simulink model "CLLLC_Plant_vLoad_V2"  (R2022a)
settings: Solver=FixedStepDiscrete  StartTime=0.0  StopTime=0.5  FixedStep=Step_Rate  RelTol=1e-3
model workspace (MAT data in the model file):
  CVI_INit = 0
  Fsw = Simulink.Signal
  Fsw.DataType = 'double'
  Fsw.Dimensions = -1
  Fsw.DimensionsMode = 'auto'
  Fsw.Complexity = 'auto'
  Fsw.SampleTime = -1
  Fsw.SamplingMode = 'auto'
  Fsw.InitialValue = 'fsw'
  L_Lim = 0.6
  fnerr = Simulink.Signal
  fnerr.DataType = 'double'
  fnerr.Dimensions = 1
  fnerr.DimensionsMode = 'Variable'
  fnerr.Complexity = 'auto'
  fnerr.SampleTime = -1
  fnerr.SamplingMode = 'auto'
  fsw = Simulink.Signal
  fsw.DataType = 'double'
  fsw.Dimensions = 1
  fsw.DimensionsMode = 'Variable'
  fsw.Complexity = 'auto'
  fsw.SampleTime = -1
  fsw.SamplingMode = 'auto'
  swit = Simulink.Signal
  swit.DataType = 'double'
  swit.Min = 0
  swit.Max = 1
  swit.Dimensions = -1
  swit.DimensionsMode = 'auto'
  swit.Complexity = 'auto'
  swit.SampleTime = -1
  swit.SamplingMode = 'auto'
  tsw = Simulink.Signal
  tsw.DataType = 'double'
  tsw.Dimensions = 1
  tsw.DimensionsMode = 'Variable'
  tsw.Complexity = 'auto'
  tsw.SampleTime = -1
  tsw.SamplingMode = 'auto'
values from neighbouring files (symbols this model uses):
  a0_cv_F = 0.01392699    [CLLLC_Plant_Parameters_vLoad_V2.m]
  a1_cv_F = -0.0060730    (= -0.006073)    [CLLLC_Plant_Parameters_vLoad_V2.m]
  a2_cv_F = 0.0    (= 0)    [CLLLC_Plant_Parameters_vLoad_V2.m]
  b1_cv_F = -1    [CLLLC_Plant_Parameters_vLoad_V2.m]
  b2_cv_F = 0.0    (= 0)    [CLLLC_Plant_Parameters_vLoad_V2.m]
  Cmd_Ref_Ctrl = round(Cmd_Ref * KVpri / VADC * ADCFS)    [CLLLC_Plant_Parameters_vLoad_V2.m]
  Control_Step_Rate = 50e-6    (= 5e-05)    [CLLLC_Plant_Parameters_vLoad_V2.m]
  Freq_Sw = 55.1e3    (= 55100)    [CLLLC_Plant_Parameters_vLoad_V2.m]
  KIout = 20e-3    (= 0.02)    [CLLLC_Plant_Parameters_vLoad_V2.m]
  KVpri = 0.0036102    [CLLLC_Plant_Parameters_vLoad_V2.m]
  KVsec = 0.00569815    [CLLLC_Plant_Parameters_vLoad_V2.m]
  Lm1 = Ln*LrP1    (= 8e-05)    [CLLLC_Plant_Parameters_vLoad_V2.m]
  n = 20.0/9.0    (= 2.22222222222)    [CLLLC_Plant_Parameters_vLoad_V2.m]
  R_series = 3    [CLLLC_Plant_Parameters_vLoad_V2.m]
  Reverse = 1    [CLLLC_Plant_Parameters_vLoad_V2.m]
  Step_Rate = 1e-7    (= 1e-07)    [CLLLC_Plant_Parameters_vLoad_V2.m]
  transformerCoupling = 0.999    [CLLLC_Plant_Parameters_vLoad_V2.m]
  Ts_Sw = floor(Fclk/Freq_Sw)    [CLLLC_Plant_Parameters_vLoad_V2.m]
libraries: fl_lib x36, nesl_utility x25, ee_lib x15, simulink x7, spsFirstOrderFilterLib x5, slpidlib x3, simulink_extras x3, eeGeneralControl x1
(part 1 of 3)
settings Model: Creator=siddharthaisukappal  LastModifiedBy=sgcesuser3
settings SolverCC: AlgebraicLoopSolver=TrustRegion
settings DataIOCC: ReturnWorkspaceOutputs=off
settings OptimizationCC: DefaultParameterBehavior=Inlined  UseDivisionForNetSlopeComputation=on  GainParamInheritBuiltInType=on  UseFloatMulNetSlope=on  InlineInvariantSignals=on  PassReuseOutputArgsAs=Individual arguments  ZeroExternalMemoryAtStartup=off  ZeroInternalMemoryAtStartup=off  NoFixptDivByZeroProtection=on  EfficientFloat2IntCast=on  LifeSpan=1  OptimizeBlockOrder=speed  DifferentSizesBufferReuse=on  EfficientTunableParamExpr=on
settings DebuggingCC: ParameterTunabilityLossMsg=error  UnconnectedInputMsg=warning  UnconnectedOutputMsg=warning  UnconnectedLineMsg=warning  SFMachineParentedDataDiag=warning
settings HardwareCC: ProdLongLongMode=on
settings SFSimCC: MATLABDynamicMemAlloc=off  CustomCodeUndefinedFunction=UseInterfaceOnly
settings RTWCC: SystemTargetFile=ert.tlc  TemplateMakefile=ert_default_tmf  GenerateReport=on  IncludeHyperlinkInReport=on  LaunchReport=on  GenerateTraceInfo=on  GenerateTraceReport=on  GenerateTraceReportSl=on  GenerateTraceReportSf=on  GenerateTraceReportEml=on  GenerateCodeMetricsReport=on  DLArmComputeVersion=19.05
settings CodeAppCC: ForceParamTrailComments=on  IgnoreCustomStorageClasses=off  OperatorAnnotations=on  SimulinkDataObjDesc=on  SFDataObjDesc=on  CustomSymbolStrGlobalVar=rt$N$M  CustomSymbolStrType=$N$M  CustomSymbolStrFcn=$N$M$F  CustomSymbolStrMacro=$N$M  InsertBlockDesc=on
settings ERTTargetCC: TargetLangStandard=C99 (ISO)  GenerateSampleERTMain=on  IncludeMdlTerminateFcn=off  CombineSignalStateStructs=on  SupportAbsoluteTime=off  SupportComplex=off  SupportContinuousTime=on  SupportNonInlinedSFcns=on  InlinedParameterPlacement=NonHierarchical  ERTCustomFileTemplate=example_file_process.tlc  ERTFilePackagingFormat=CompactWithDataFile
settings SimscapeCC: SimscapeLogDataHistory=20000

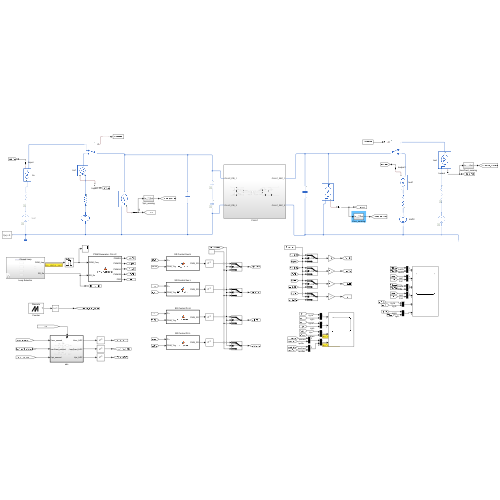
[thumbnail: Simulink's stored preview of the top-level diagram]
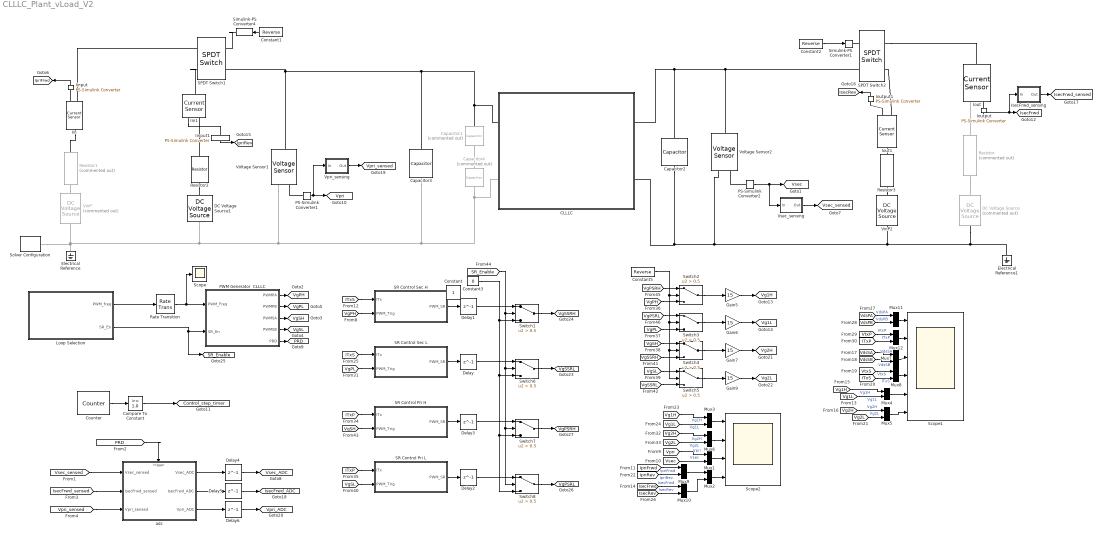
== system CLLLC_Plant_vLoad_V2 ==
  CLLLC : Subsystem
  Capacitor1 : fl_lib/Electrical/Electrical Elements/Capacitor  Commented=on  c=2800e-6 F  r=0.0496 Ohm  g=0 1/Ohm  i_specify=off  i_priority=None  i=0 A  i_nominal_specify=off  i_nominal_unit=A  i_nominal_value=1  v_specify=off  v_priority=None  v=390 V  v_nominal_specify=off  v_nominal_unit=V  v_nominal_value=1  vc_specify=on  vc_priority=High  vc=403 V  vc_nominal_specify=off  vc_nominal_unit=V  vc_nominal_value=1
      settings: SourceProductBaseCode=PW,SS,VE
  Capacitor2 : fl_lib/Electrical/Electrical Elements/Capacitor  c=50e-6 F  r=9.5e-3 Ohm  g=0 1/Ohm  i_specify=off  i_priority=None  i=0 A  i_nominal_specify=off  i_nominal_unit=A  i_nominal_value=1  v_specify=off  v_priority=None  v=400 V  v_nominal_specify=off  v_nominal_unit=V  v_nominal_value=1  vc_specify=on  vc_priority=High  vc=200 V  vc_nominal_specify=off  vc_nominal_unit=V  vc_nominal_value=1
      settings: SourceProductBaseCode=PW,SS,VE
  Capacitor3 : fl_lib/Electrical/Electrical Elements/Capacitor  c=88e-6 F  r=1.1e-3 Ohm  g=0 1/Ohm  i_specify=off  i_priority=None  i=0 A  i_nominal_specify=off  i_nominal_unit=A  i_nominal_value=1  v_specify=off  v_priority=None  v=780 V  v_nominal_specify=off  v_nominal_unit=V  v_nominal_value=1  vc_specify=off  vc_priority=High  vc=806 V  vc_nominal_specify=off  vc_nominal_unit=V  vc_nominal_value=1
      settings: SourceProductBaseCode=PW,SS,VE
  Capacitor4 : fl_lib/Electrical/Electrical Elements/Capacitor  Commented=on  c=2800e-6 F  r=0.0496 Ohm  g=0 1/Ohm  i_specify=off  i_priority=None  i=0 A  i_nominal_specify=off  i_nominal_unit=A  i_nominal_value=1  v_specify=off  v_priority=None  v=390 V  v_nominal_specify=off  v_nominal_unit=V  v_nominal_value=1  vc_specify=on  vc_priority=High  vc=403 V  vc_nominal_specify=off  vc_nominal_unit=V  vc_nominal_value=1
      settings: SourceProductBaseCode=PW,SS,VE
  Compare To Constant : simulink/Logic and Bit Operations/Compare To Constant  relop=>=  const=1.0  OutDataTypeStr=boolean
  Constant1 : Constant  Value=Reverse
  Constant2 : Constant  Value=Reverse
  Constant3 : Constant  Value=0
  Constant5 : Constant  Value=Reverse
  Counter : eeGeneralControl/Counter  CarrCount=Up  Range=[0 1]  Tper=Control_Step_Rate  Tdelay=0  Ts=Step_Rate
      settings: SourceProductBaseCode=PS
  DC Voltage Source : fl_lib/Electrical/Electrical Sources/DC Voltage Source  Commented=on  v0=V_Load V
      settings: SourceProductBaseCode=PW,SS,VE
  DC Voltage Source1 : fl_lib/Electrical/Electrical Sources/DC Voltage Source  v0=V_Load V
      settings: SourceProductBaseCode=PW,SS,VE
  Delay{,1..5} (6 alike) : Delay  DelayLength=1
  Delay6 : Delay  DelayLength=1  InitialCondition=0
  Electrical Reference : fl_lib/Electrical/Electrical Elements/Electrical Reference
      settings: SourceProductBaseCode=PW,SS,VE
  Electrical Reference1 : fl_lib/Electrical/Electrical Elements/Electrical Reference
      settings: SourceProductBaseCode=PW,SS,VE
  Gain{5..7,9} (4 alike) : Gain  Gain=15
  Iin : fl_lib/Electrical/Electrical Sensors/Current Sensor
      settings: SourceProductBaseCode=PW,SS,VE
  Iin1 : fl_lib/Electrical/Electrical Sensors/Current Sensor
      settings: SourceProductBaseCode=PW,SS,VE
  Iinput : nesl_utility/PS-Simulink Converter  PhysicalDomain=network_engine_domain  SubClassName=ps_output  LeftPortType=input  RightPortType=output  PseudoPeriodic=off  Frequencies=[]  VectorFormat=1-D array  Unit=A  AffineConversion=off
      settings: SourceProductBaseCode=SS,PW,VE
  Iinput1 : nesl_utility/PS-Simulink Converter  PhysicalDomain=network_engine_domain  SubClassName=ps_output  LeftPortType=input  RightPortType=output  PseudoPeriodic=off  Frequencies=[]  VectorFormat=1-D array  Unit=A  AffineConversion=off
      settings: SourceProductBaseCode=SS,PW,VE
  Iout : fl_lib/Electrical/Electrical Sensors/Current Sensor
      settings: SourceProductBaseCode=PW,SS,VE
  Iout1 : fl_lib/Electrical/Electrical Sensors/Current Sensor
      settings: SourceProductBaseCode=PW,SS,VE
  Ioutput : nesl_utility/PS-Simulink Converter  PhysicalDomain=network_engine_domain  SubClassName=ps_output  LeftPortType=input  RightPortType=output  PseudoPeriodic=off  Frequencies=[]  VectorFormat=1-D array  Unit=A  AffineConversion=off
      settings: SourceProductBaseCode=SS,PW,VE
  Ioutput1 : nesl_utility/PS-Simulink Converter  PhysicalDomain=network_engine_domain  SubClassName=ps_output  LeftPortType=input  RightPortType=output  PseudoPeriodic=off  Frequencies=[]  VectorFormat=1-D array  Unit=A  AffineConversion=off
      settings: SourceProductBaseCode=SS,PW,VE
  IsecFrwd_sensing : Subsystem
  Loop Selection : Subsystem  Variant=on
  Mux{1..12} (12 alike) : Mux  Inputs=2
  PS-Simulink Converter1 : nesl_utility/PS-Simulink Converter  PhysicalDomain=network_engine_domain  SubClassName=ps_output  LeftPortType=input  RightPortType=output  PseudoPeriodic=off  Frequencies=[]  VectorFormat=1-D array  Unit=V  AffineConversion=off
      settings: SourceProductBaseCode=SS,PW,VE
  PS-Simulink Converter2 : nesl_utility/PS-Simulink Converter  PhysicalDomain=network_engine_domain  SubClassName=ps_output  LeftPortType=input  RightPortType=output  PseudoPeriodic=off  Frequencies=[]  VectorFormat=1-D array  Unit=V  AffineConversion=off
      settings: SourceProductBaseCode=SS,PW,VE
  PWM Generator  CLLLC : MATLAB Function  TreatAsAtomicUnit=on  SystemSampleTime=Step_Rate
  Rate Transition : RateTransition  InitialCondition=240000
  Resistor : ee_lib/Passive/Resistor  Commented=on  R=R_series Ohm  enable_R_tol=0  R_tol=5  tol_distribution=1  nSigma=4  enable_operating_limits=0  operating_limit_action=2  max_working_voltage=100 V  power_rating=1 W  enable_faults=0  fault_action=1  R_faulted=inf Ohm  enable_temporal_fault=0  t_fault=1 s  enable_behavioral_fault=0  max_permissible_current=1 A  t_fail_on_current=1 s  noise_mode=0  sample_time=1e-3 s  repeatability=1  auto_seed=913116633  user_seed=0  Tdevice=25 degC  power_derating_T1=70 degC  power_derating_T2=155 degC  operating_temperature_range_vec=[-50, 150] degC  alpha=3.93e-3 1/K  Tmeas=25 degC  thermal_mass=100 J/K  temperature_specify=off  temperature_priority=High  temperature=298.15 K  temperature_nominal_specify=off  temperature_nominal_unit=K  temperature_nominal_value=1
  Resistor1 : ee_lib/Passive/Resistor  Commented=on  R=0.1 Ohm  enable_R_tol=0  R_tol=5  tol_distribution=1  nSigma=4  enable_operating_limits=0  operating_limit_action=2  max_working_voltage=100 V  power_rating=1 W  enable_faults=0  fault_action=1  R_faulted=inf Ohm  enable_temporal_fault=0  t_fault=1 s  enable_behavioral_fault=0  max_permissible_current=1 A  t_fail_on_current=1 s  noise_mode=0  sample_time=1e-3 s  repeatability=1  auto_seed=2493270049  user_seed=0  Tdevice=25 degC  power_derating_T1=70 degC  power_derating_T2=155 degC  operating_temperature_range_vec=[-50, 150] degC  alpha=3.93e-3 1/K  Tmeas=25 degC  thermal_mass=100 J/K  temperature_specify=off  temperature_priority=High  temperature=298.15 K  temperature_nominal_specify=off  temperature_nominal_unit=K  temperature_nominal_value=1
  Resistor2 : ee_lib/Passive/Resistor  R=R_series Ohm  enable_R_tol=0  R_tol=5  tol_distribution=1  nSigma=4  enable_operating_limits=0  operating_limit_action=2  max_working_voltage=100 V  power_rating=1 W  enable_faults=0  fault_action=1  R_faulted=inf Ohm  enable_temporal_fault=0  t_fault=1 s  enable_behavioral_fault=0  max_permissible_current=1 A  t_fail_on_current=1 s  noise_mode=0  sample_time=1e-3 s  repeatability=1  auto_seed=3499211588  user_seed=0  Tdevice=25 degC  power_derating_T1=70 degC  power_derating_T2=155 degC  operating_temperature_range_vec=[-50, 150] degC  alpha=3.93e-3 1/K  Tmeas=25 degC  thermal_mass=100 J/K  temperature_specify=off  temperature_priority=High  temperature=298.15 K  temperature_nominal_specify=off  temperature_nominal_unit=K  temperature_nominal_value=1
  Resistor3 : ee_lib/Passive/Resistor  R=0.1 Ohm  enable_R_tol=0  R_tol=5  tol_distribution=1  nSigma=4  enable_operating_limits=0  operating_limit_action=2  max_working_voltage=100 V  power_rating=1 W  enable_faults=0  fault_action=1  R_faulted=inf Ohm  enable_temporal_fault=0  t_fault=1 s  enable_behavioral_fault=0  max_permissible_current=1 A  t_fail_on_current=1 s  noise_mode=0  sample_time=1e-3 s  repeatability=1  auto_seed=3890346746  user_seed=0  Tdevice=25 degC  power_derating_T1=70 degC  power_derating_T2=155 degC  operating_temperature_range_vec=[-50, 150] degC  alpha=3.93e-3 1/K  Tmeas=25 degC  thermal_mass=100 J/K  temperature_specify=off  temperature_priority=High  temperature=298.15 K  temperature_nominal_specify=off  temperature_nominal_unit=K  temperature_nominal_value=1
  SPDT Switch1 : ee_lib/Switches & Breakers/SPDT Switch  R_closed=0.01 Ohm  G_open=1e-6 S  Threshold=0.5 V  Width=0 V  model_dynamics=0  t_on=1e-3 s  t_off=1e-3 s  initial_vT=0 V
      settings: SourceProductBaseCode=PS
  SPDT Switch2 : ee_lib/Switches & Breakers/SPDT Switch  R_closed=0.01 Ohm  G_open=1e-6 S  Threshold=0.5 V  Width=0 V  model_dynamics=0  t_on=1e-3 s  t_off=1e-3 s  initial_vT=0 V
      settings: SourceProductBaseCode=PS
  SR Control Pri H : MATLAB Function  TreatAsAtomicUnit=on  SystemSampleTime=Step_Rate
  SR Control Pri L : MATLAB Function  TreatAsAtomicUnit=on  SystemSampleTime=Step_Rate
  SR Control Sec H : MATLAB Function  TreatAsAtomicUnit=on  SystemSampleTime=Step_Rate
  SR Control Sec L : MATLAB Function  TreatAsAtomicUnit=on  SystemSampleTime=Step_Rate
  Scope : Scope
  Scope1 : Scope  NumInputPorts=6
  Scope2 : Scope  NumInputPorts=4
  Simulink-PS Converter1 : nesl_utility/Simulink-PS Converter  PhysicalDomain=network_engine_domain  SubClassName=ps_input  LeftPortType=input  RightPortType=output  PseudoPeriodic=off  Frequencies=[]  NoiseDistribution=none  NoiseParameters=[]  Unit=1  AffineConversion=off  FilteringAndDerivatives=provide  SimscapeFilterOrder=1  InputFilterTimeConstant=0.001  UdotUserProvided=0
      settings: SourceProductBaseCode=SS,PW,VE
  Simulink-PS Converter4 : nesl_utility/Simulink-PS Converter  PhysicalDomain=network_engine_domain  SubClassName=ps_input  LeftPortType=input  RightPortType=output  PseudoPeriodic=off  Frequencies=[]  NoiseDistribution=none  NoiseParameters=[]  Unit=1  AffineConversion=off  FilteringAndDerivatives=provide  SimscapeFilterOrder=1  InputFilterTimeConstant=0.001  UdotUserProvided=0
      settings: SourceProductBaseCode=SS,PW,VE
  Solver Configuration : nesl_utility/Solver Configuration  PhysicalDomain=network_engine_domain  SubClassName=solver  LeftPortType=input  RightPortType=generic  Tones=[]  Harmonics=[]  SimulateNoise=off  Profile=off  UseLocalSampling=off  EnableSwitchedLinearOptims=on  FrequencyDomain=off  UseCCode=off  RelTol=0.001  AbsTol=1e-06  MinStep=1e-09  ToWorkspace=off  RevertToSquareIcSolve=off  NumHomotopyIterations=100  PhasorMode=off  PhasorModeNumHarmonics=1  IndexReductionMethod=DerivativeReplacement  DoDC=off  ResidualTolerance=1e-07  UseLocalSolver=on  LocalSolverChoice=NE_BACKWARD_EULER_ADVANCER  LocalSolverSampleTime=Step_Rate  DoFixedCost=off  MaxNonlinIter=3  MaxModeIter=2  ComputeImpulses=off  ImpulseIterations=2  LinearAlgebra=auto  LinearAlgebraNumThread=0  EquationFormulation=NE_TIME_EF  DelaysMemoryBudget=1024  AutomaticFiltering=on  FilteringTimeConstant=0.001  PartitionStorageMethod=AS_NEEDED  PartitionMemoryBudget=1024  PartitionMethod=FAST
      settings: SourceProductBaseCode=SS,PW,VE
  Switch{1..8} (8 alike) : Switch  Criteria=u2 > Threshold  Threshold=0.5  SaturateOnIntegerOverflow=off  InputSameDT=off
  VinP : fl_lib/Electrical/Electrical Sources/DC Voltage Source  Commented=on  v0=V_Input V
      settings: SourceProductBaseCode=PW,SS,VE
  VinP2 : fl_lib/Electrical/Electrical Sources/DC Voltage Source  v0=V_Input V
      settings: SourceProductBaseCode=PW,SS,VE
  Voltage Sensor1 : fl_lib/Electrical/Electrical Sensors/Voltage Sensor
      settings: SourceProductBaseCode=PW,SS,VE
  Voltage Sensor2 : fl_lib/Electrical/Electrical Sensors/Voltage Sensor
      settings: SourceProductBaseCode=PW,SS,VE
  Vpri_sensing : Subsystem
  Vsec_sensing : Subsystem
  adc : Subsystem
  Constant : Constant  IOType=siggen
  tag scope: Control_step_timer=global, IpriFrwd=global, IpriRev=global, IsecFrwd=global, IsecFrwd_ADC=global, IsecFrwd_sensed=global, IsecRev=global, PRD=global, SR_Enable=global, Vg1H=global, Vg1L=global, Vg2H=global, Vg2L=global, VgPH=global, VgPL=global, VgPSRH=global, VgPSRL=global, VgSH=global, VgSL=global, VgSSRH=global, VgSSRL=global, Vpri=global, Vpri_ADC=global, Vpri_sensed=global, Vsec=global, Vsec_ADC=global, Vsec_sensed=global
  wires:
  [Vg1H] -> Mux3/1  "Vg1H"
  Mux9/1 -> Mux2/1
  [Vg2H] -> Mux6/1  "Vg2H"
  Mux3/1 -> Scope2/1
  Mux2/1 -> Scope2/4
  Mux6/1 -> Scope2/2
  PWM Generator  CLLLC/1(PWMPA) -> [VgPH]
  Mux1/1 -> Scope2/3
  [Vsec] -> Mux1/2  "Vsec"
  [Vg2L] -> Mux6/2  "Vg2L"
  [Vpri] -> Mux1/1  "Vpri"
  PWM Generator  CLLLC/3(PWMSA) -> [VgSH]
  [Vg1L] -> Mux3/2  "Vg1L"
  PWM Generator  CLLLC/4(PWMSB) -> [VgSL]
  PWM Generator  CLLLC/2(PWMPB) -> [VgPL]
  Iinput/1 -> [IpriFrwd]
  PS-Simulink Converter2/1 -> Vsec_sensing/1(In), [Vsec]
  Ioutput/1 -> IsecFrwd_sensing/1(In), [IsecFrwd]
  [VdsSB] -> Mux7/2  "VdsSB"
  [Vg1H] -> Mux4/1  "Vg1H"
  Mux5/1 -> Scope1/6
  [VdsSA] -> Mux7/1  "VdsSA"
  [Vg2L] -> Mux5/2  "Vg2L"
  Constant1/1 -> Simulink-PS Converter4/1
  Constant2/1 -> Simulink-PS Converter1/1
  Iinput1/1 -> [IpriRev]
  [IpriFrwd] -> Mux9/1  "IpriFrwd"
  [IpriRev] -> Mux9/2  "IpriRev"
  [IsecFrwd] -> Mux10/1  "IsecFrwd"
  Mux10/1 -> Mux2/2
  Ioutput1/1 -> [IsecRev]
  [IsecRev] -> Mux10/2  "IsecRev"
  Mux4/1 -> Scope1/5
  Mux8/1 -> Scope1/4
  Mux7/1 -> Scope1/3
  Mux11/1 -> Scope1/1
  Mux12/1 -> Scope1/2
  [VdsPA] -> Mux11/1  "VdsPA"
  [VdsPB] -> Mux11/2  "VdsPB"
  Switch2/1 -> Gain5/1
  Gain5/1 -> [Vg1H]
  [VgPH] -> Switch2/3
  [VgPL] -> Switch3/3
  Gain6/1 -> [Vg1L]
  Switch3/1 -> Gain6/1
  Switch4/1 -> Gain7/1
  Gain7/1 -> [Vg2H]
  Gain9/1 -> [Vg2L]
  Switch5/1 -> Gain9/1
  Constant5/1 -> Switch5/2, Switch4/2, Switch3/2, Switch2/2
  [VgSH] -> Switch4/1
  [VgSL] -> Switch5/1
  [VgSSRH] -> Switch4/3
  [VgSSRL] -> Switch5/3
  Delay1/1 -> Switch1/1
  Switch1/1 -> [VgSSRH]
  Switch6/1 -> [VgSSRL]
  Delay/1 -> Switch6/1
  Delay2/1 -> Switch8/1
  Constant3/1 -> Switch7/3, Switch8/3, Switch6/3, Switch1/3
  Delay3/1 -> Switch7/1
  [SR_Enable] -> Switch7/2, Switch8/2, Switch6/2, Switch1/2
  Switch7/1 -> [VgPSRH]
  Switch8/1 -> [VgPSRL]
  [VgPSRL] -> Switch3/1
  [VgPSRH] -> Switch2/1
  SR Control Sec H/1(PWM_SR) -> Delay1/1
  [VgPH] -> SR Control Sec H/2(PWM_Trig)
  [ITxS] -> SR Control Sec H/1(ITx)
  [ITxS] -> SR Control Sec L/1(ITx)
  [VgPL] -> SR Control Sec L/2(PWM_Trig)
  SR Control Sec L/1(PWM_SR) -> Delay/1
  SR Control Pri L/1(PWM_SR) -> Delay2/1
  [VgSL] -> SR Control Pri L/2(PWM_Trig)
  [ITxP] -> SR Control Pri L/1(ITx)
  [ITxP] -> SR Control Pri H/1(ITx)
  [VgSH] -> SR Control Pri H/2(PWM_Trig)
  SR Control Pri H/1(PWM_SR) -> Delay3/1
  Rate Transition/1 -> Scope/1, PWM Generator  CLLLC/1(PWM_Freq)
  Loop Selection/1(PWM_freq) -> Rate Transition/1
  Loop Selection/2(SR_En) -> [SR_Enable], PWM Generator  CLLLC/2(SR_En)
  [Vg1L] -> Mux4/2  "Vg1L"
  [Vg2H] -> Mux5/1  "Vg2H"
  [VtxS] -> Mux8/1  "VtxS"
  [ITxS] -> Mux8/2  "ITxS"
  [ITxP] -> Mux12/2  "ITxP"
  [VtxP] -> Mux12/1  "VtxP"
  Vsec_sensing/1(Out) -> [Vsec_sensed]
  adc/1(Vsec_ADC) -> Delay4/1
  PWM Generator  CLLLC/5(PRD) -> [PRD]
  [PRD] -> adc/Trigger
  [Vsec_sensed] -> adc/1(Vsec_sensed)
  Delay4/1 -> [Vsec_ADC]
  Counter/1 -> Compare To Constant/1
  Compare To Constant/1 -> [Control_step_timer]
  IsecFrwd_sensing/1(Out) -> [IsecFrwd_sensed]
  [IsecFrwd_sensed] -> adc/2(IsecFrwd_sensed)
  adc/2(IsecFrwd_ADC) -> Delay5/1
  Delay5/1 -> [IsecFrwd_ADC]
  PS-Simulink Converter1/1 -> [Vpri], Vpri_sensing/1(In)
  Vpri_sensing/1(Out) -> [Vpri_sensed]
  [Vpri_sensed] -> adc/3(Vpri_sensed)
  adc/3(Vpri_ADC) -> Delay6/1
  Delay6/1 -> [Vpri_ADC]
  connections:
  Capacitor4/RConn1 -- Capacitor3/RConn1 -- Voltage Sensor1/RConn2 -- DC Voltage Source1/RConn1 -- Electrical Reference/LConn1 -- Solver Configuration/RConn1 -- VinP/RConn1 -- CLLLC/LConn2
  Iin/RConn1 -- Iinput/LConn1
  PS-Simulink Converter1/LConn1 -- Voltage Sensor1/RConn1
  Iout/RConn1 -- Ioutput/LConn1
  PS-Simulink Converter2/LConn1 -- Voltage Sensor2/RConn1
  Simulink-PS Converter4/RConn1 -- SPDT Switch1/LConn1
  Iin/RConn2 -- SPDT Switch1/RConn1
  Simulink-PS Converter1/RConn1 -- SPDT Switch2/LConn1
  Iin/LConn1 -- Resistor1/LConn1
  Iin1/RConn1 -- Iinput1/LConn1
  SPDT Switch1/RConn2 -- Iin1/LConn1
  Resistor2/LConn1 -- Iin1/RConn2
  SPDT Switch2/RConn1 -- Iout/LConn1
  Iout1/RConn1 -- Ioutput1/LConn1
  Iout1/RConn2 -- SPDT Switch2/RConn2
  Voltage Sensor2/LConn1 -- CLLLC/RConn1 -- Capacitor2/LConn1 -- SPDT Switch2/LConn2
  Capacitor4/LConn1 -- Capacitor1/RConn1
  Resistor/RConn1 -- DC Voltage Source/LConn1
  Resistor/LConn1 -- Iout/RConn2
  Iout1/LConn1 -- Resistor3/LConn1
  Capacitor3/LConn1 -- Capacitor1/LConn1 -- CLLLC/LConn1 -- Voltage Sensor1/LConn1 -- SPDT Switch1/LConn2
  Voltage Sensor2/RConn2 -- Electrical Reference1/LConn1 -- DC Voltage Source/RConn1 -- VinP2/RConn1 -- CLLLC/RConn2 -- Capacitor2/RConn1
  Resistor1/RConn1 -- VinP/LConn1
  Resistor2/RConn1 -- DC Voltage Source1/LConn1
  Resistor3/RConn1 -- VinP2/LConn1
